simulink model "Conventional_Buck_DCMen_PractPSU_OL"  (R2017b)
settings: Solver=ode1  StartTime=0.0  StopTime=2e-3  FixedStep=Ts  RelTol=1e-3
PostLoadFcn:
  | , if any(exist('dsrtsu_mdlpostloadfcn', 'file') == [2, 3, 6]), try dsrtsu_mdlpostloadfcn('Execute', bdroot); catch fprintf('Error in PostLoadFcn (dsrtsu_mdlpostloadfcn) for model "%s":\n %s\n', bdroot, lasterr); end, end,
  | init_conventional_buck;
InitFcn:
  | init_conventional_buck;
values from neighbouring files (symbols this model uses):
  DCM_en = 1    [init_conventional_buck_lec13.m]
  IL_transient_en = 0    [init_conventional_buck_lec13.m]
  Ts = 10e-9    (= 1e-08)    [init_conventional_buck.m]    (also in init_conventional_buck_lec13.m)
  Vin = 12    [init_conventional_buck.m]    (also in init_conventional_buck_lec13.m)
  Vmax = 10    [init_conventional_buck.m]    (also in init_conventional_buck_lec13.m)
  Vref = 3.3    [init_conventional_buck.m]    (also in init_conventional_buck_lec13.m = 1)
libraries: simulink x3
Description:
  | Standard RTI1005 template.
  | Supported MATLAB version:  R2017b.
settings Model: Tag=RTI1005  DSRTSU_INTERNAL_RTI_VER=540  DSRTSU_INTERNAL_RTI_TYPE=rti1005  RTICANMMDATA=struct('GeneralSetupData',struct('modelroot','C:\Projects\Simulink\PE_1\w3\lec13','generalsettings',struct('filesettings',struct('destfolder',struct('Name','RTICANMM_FILES','Check',1),'buildfolder',struct('Name','.','Check',1),'AbsDestfolder',struct('Name','C:\Projects\Simulink\PE_1\w3\lec13\RTICANMM_FILES'),'AbsBuildfolder',struct('Name','C:\Projects\Simulink\PE_1\w3\lec13'))),'options',struct('addpaths',1,'rmpaths',1,'addtrcexclusion',logical(1),'cannavigator',struct('checkmonitoring',0),'show_usrtrc',0,'use_usrtrc',0),'advanced',struct('options',ones(1,100)),'MPSetup',{{}},'RTI',struct('Type','RTI1005','Ver','7.12','Date','02-May-2019'),'modelname','Conventional_Buck_DCMen_PractPSU_OL','block','Conventional_Buck_DCMen_PractPSU_OL'))  DSRTSU_INTERNAL_RTIFPGA=130  Creator=CA72672  LastModifiedBy=CA72672
settings OptimizationCC: BlockReduction=off  OptimizeBlockIOStorage=off  BufferReuse=off  GlobalBufferReuse=off  ExpressionFolding=off  LocalBlockOutputs=off
settings HardwareCC: ProdBitPerPointer=32  ProdBitPerSizeT=32  ProdBitPerPtrDiffT=32  ProdLargestAtomicInteger=Integer  ProdEndianess=BigEndian  ProdWordSize=32  ProdHWDeviceType=Custom Processor->Custom  TargetIntDivRoundTo=Zero  TargetEndianess=BigEndian  TargetHWDeviceType=Custom Processor->Custom
settings SFSimCC: MATLABDynamicMemAlloc=off
settings RTWCC: SystemTargetFile=rti1005.tlc  MakeCommand=make_rti  TemplateMakefile=rti1005.tmf  Description=dSPACE DS1005 Hardware Platform
settings CodeAppCC: StateflowObjectComments=on
settings STFCustomTargetCC: ParMdlRefBuildCompliant=on  MatFileLogging=on  GRTInterface=off  SystemTargetFile=rti1005.tlc
settings GRTTargetCC: TargetLangStandard=C89/C90 (ANSI)  CompOptLevelCompliant=off  ConcurrentExecutionCompliant=off  CombineOutputUpdateFcns=off  CPPClassGenCompliant=off  UseToolchainInfoCompliant=off
settings ConfigComp: CovMetricSettings=dswe

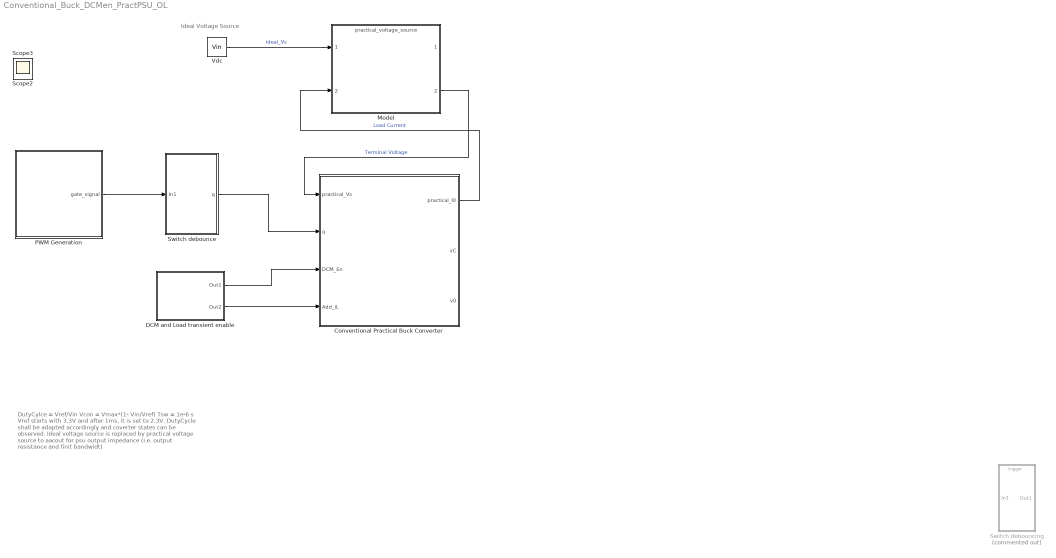
== system Conventional_Buck_DCMen_PractPSU_OL ==
  note: Ideal Voltage Source
  note: DutyCylce = Vref/Vin
      |
      | Vcon = Vmax*(1- Vin/Vref)
      |
      | Tsw = 1e-6 s
      |
      | Vref starts with 3.3V and after 1ms, it is set to 2.3V.
      | DutyCycle shall be adapted accordingly and coverter states can be observed.
      |
      | Ideal voltage source is replaced by practical voltage source to aacout for psu output impedance (i.e. output resistance and finit bandwidt)
  Conventional Practical Buck Converter : Subsystem
  DCM and Load transient enable : Subsystem
  Model : ModelReference  ModelNameDialog=practical_voltage_source.slx  SimulationMode=Normal  ModelReferenceVersion=1.12
  PWM Generation : Subsystem
  Switch debounce : Subsystem
  Switch debouncing : Subsystem  Commented=on  TreatAsAtomicUnit=on
  Vdc : Constant  Value=Vin
  Scope2 : Scope
  Scope3 : Scope
  wires:
  Model/2 -> Conventional Practical Buck Converter/1(practical_Vs)  "Terminal Voltage"
  Vdc/1 -> Model/1  "ideal_Vs"
  PWM Generation/1(gate_signal) -> Switch debounce/1(In1)
  Conventional Practical Buck Converter/1(practical_I0) -> Model/2  "Load Current"
  Switch debounce/1(q) -> Conventional Practical Buck Converter/2(q)
  DCM and Load transient enable/1(Out1) -> Conventional Practical Buck Converter/3(DCM_En)
  DCM and Load transient enable/2(Out2) -> Conventional Practical Buck Converter/4(Add_iL)

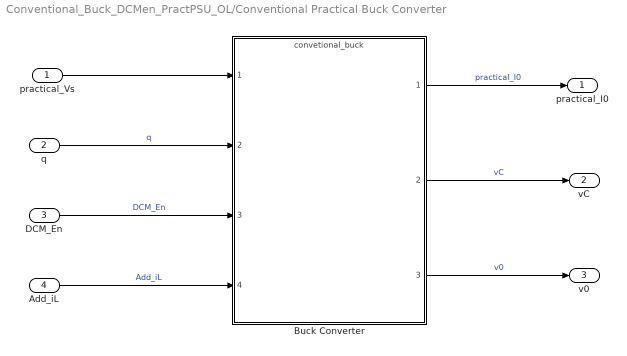
== system Conventional_Buck_DCMen_PractPSU_OL/Conventional Practical Buck Converter ==
  practical_Vs : Inport
  q : Inport  Port=2
  DCM_En : Inport  Port=3
  Add_iL : Inport  Port=4
  Buck Converter : ModelReference  ModelNameDialog=convetional_buck.slx  SimulationMode=Normal  ModelReferenceVersion=1.35
  practical_I0 : Outport
  vC : Outport  Port=2
  v0 : Outport  Port=3
  wires:
  practical_Vs/1 -> Buck Converter/1
  DCM_En/1 -> Buck Converter/3  "DCM_En"
  Add_iL/1 -> Buck Converter/4  "Add_iL"
  Buck Converter/2 -> vC/1  "vC"
  Buck Converter/1 -> practical_I0/1  "practical_I0"
  Buck Converter/3 -> v0/1  "v0"
  q/1 -> Buck Converter/2  "q"

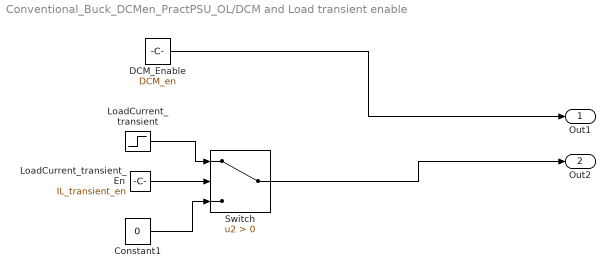
== system Conventional_Buck_DCMen_PractPSU_OL/DCM and Load transient enable ==
  Constant1 : Constant  Value=0
  DCM_Enable : Constant  Value=DCM_en  OutDataTypeStr=boolean
  LoadCurrent_transient : Step  Time=1.5e-3  Before=2  After=4
  LoadCurrent_transient_En : Constant  Value=IL_transient_en  OutDataTypeStr=boolean
  Switch : Switch  Criteria=u2 > Threshold
  Out1 : Outport
  Out2 : Outport  Port=2
  wires:
  Switch/1 -> Out2/1
  DCM_Enable/1 -> Out1/1
  Constant1/1 -> Switch/3
  LoadCurrent_transient_En/1 -> Switch/2
  LoadCurrent_transient/1 -> Switch/1

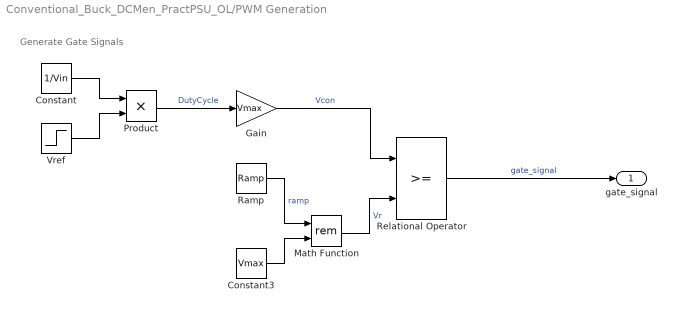
== system Conventional_Buck_DCMen_PractPSU_OL/PWM Generation ==
  note: Generate Gate Signals
  Constant : Constant  Value=1/Vin
  Constant3 : Constant  Value=Vmax
  Gain : Gain  Gain=Vmax
  Math Function : Math  Operator=rem  SaturateOnIntegerOverflow=on
  Product : Product
  Ramp : simulink/Sources/Ramp  slope=Vmax/Tsw  start=0  X0=0
  Relational Operator : RelationalOperator  OutDataTypeStr=boolean  RndMeth=Simplest
  Vref : Step  Time=1.05e-3  Before=Vref  After=Vref-1
  gate_signal : Outport
  wires:
  Constant/1 -> Product/1
  Vref/1 -> Product/2
  Product/1 -> Gain/1  "DutyCycle"
  Constant3/1 -> Math Function/2
  Gain/1 -> Relational Operator/1  "Vcon"
  Ramp/1 -> Math Function/1  "ramp"
  Math Function/1 -> Relational Operator/2  "Vr"
  Relational Operator/1 -> gate_signal/1  "gate_signal"

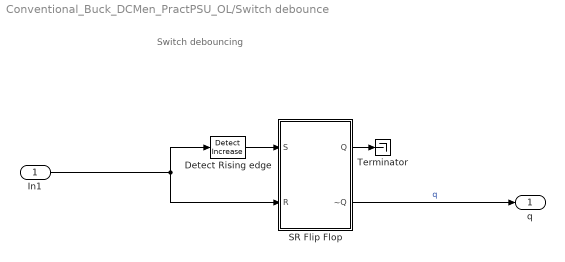
== system Conventional_Buck_DCMen_PractPSU_OL/Switch debounce ==
  note: Switch debouncing
  In1 : Inport
  Detect Rising edge : simulink/Logic and Bit Operations/Detect Increase  vinit=0.0  OutDataTypeStr=boolean
  SR Flip Flop : Subsystem
  Terminator : Terminator
  q : Outport
  wires:
  Detect Rising edge/1 -> SR Flip Flop/1(S)
  SR Flip Flop/2(~Q) -> q/1  "q"
  SR Flip Flop/1(Q) -> Terminator/1
  In1/1 -> SR Flip Flop/2(R), Detect Rising edge/1

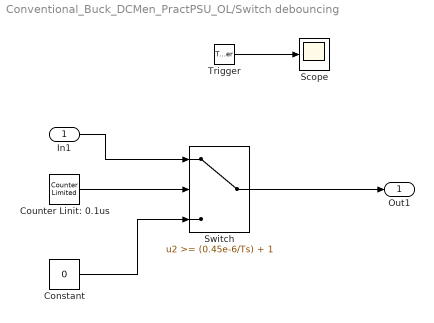
== system Conventional_Buck_DCMen_PractPSU_OL/Switch debouncing ==
  In1 : Inport
  Trigger : TriggerPort  VariantControl=Variant  ShowOutputPort=on  PortDimensions=1
  Constant : Constant  Value=0
  Counter Linit: 0.1us : simulink/Sources/Counter Limited  uplimit=(0.45e-6/Ts) + 1  tsamp=-1
  Scope : Scope
  Switch : Switch  Threshold=(0.45e-6/Ts) + 1
  Out1 : Outport
  wires:
  In1/1 -> Switch/1
  Switch/1 -> Out1/1
  Counter Linit: 0.1us/1 -> Switch/2
  Constant/1 -> Switch/3
  Trigger/1 -> Scope/1

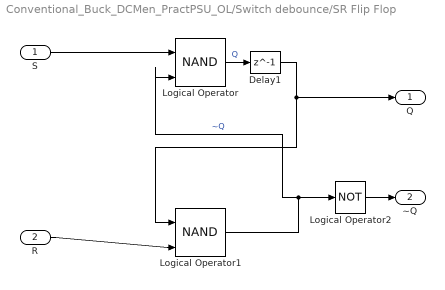
== system Conventional_Buck_DCMen_PractPSU_OL/Switch debounce/SR Flip Flop ==
  S : Inport
  R : Inport  Port=2
  Delay1 : Delay  DelayLength=1
  Logical Operator : Logic  Operator=NAND  IconShape=distinctive  AllPortsSameDT=off  OutDataTypeStr=boolean
  Logical Operator1 : Logic  Operator=NAND  IconShape=distinctive  AllPortsSameDT=off  OutDataTypeStr=boolean
  Logical Operator2 : Logic  Operator=NOT  IconShape=distinctive  AllPortsSameDT=off  OutDataTypeStr=boolean
  Q : Outport
  ~Q : Outport  Port=2
  wires:
  Delay1/1 -> Q/1, Logical Operator1/1
  S/1 -> Logical Operator/1
  R/1 -> Logical Operator1/2
  Logical Operator/1 -> Delay1/1  "Q"
  Logical Operator1/1 -> Logical Operator2/1, Logical Operator/2  "~Q"
  Logical Operator2/1 -> ~Q/1
